simulink model "Simulink_drone_BO"  (R2025b)
settings: Solver=FixedStepAuto  StartTime=0.0  StopTime=10.0  FixedStep=dt_realtime  RelTol=1e-3
undefined symbols (not defined in the file): bool, dt_realtime, sysBO, x_init
libraries: sim3dlib x1, uavsim3dlib x1, aerolibanimutils x1
settings Model: Creator=pierr  LastModifiedBy=pierr

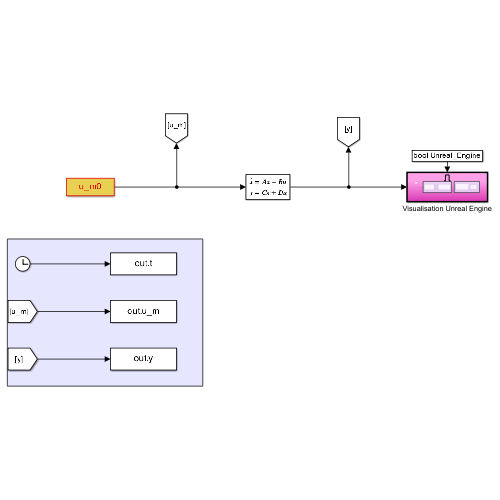
[thumbnail: Simulink's stored preview of the top-level diagram]
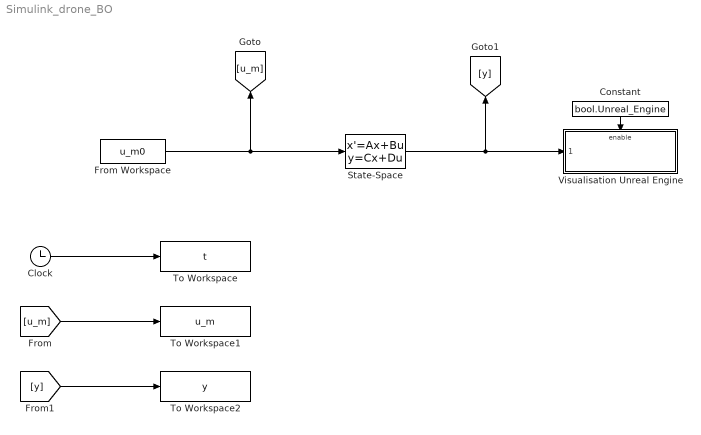
== system Simulink_drone_BO ==
  Clock : Clock
  Constant : Constant  Value=bool.Unreal_Engine
  From Workspace : FromWorkspace  VariableName=u_m0
  State-Space : StateSpace  A=sysBO.A  B=sysBO.B  C=sysBO.C  D=sysBO.D  InitialCondition=x_init
  To Workspace : ToWorkspace  VariableName=t  SaveFormat=Timeseries  SampleTime=-1
  To Workspace1 : ToWorkspace  VariableName=u_m  SaveFormat=Timeseries  SampleTime=-1
  To Workspace2 : ToWorkspace  VariableName=y  SaveFormat=Timeseries  SampleTime=-1
  Visualisation Unreal Engine : Subsystem
  wires:
  From Workspace/1 -> [u_m], State-Space/1
  Clock/1 -> To Workspace/1
  [u_m] -> To Workspace1/1
  State-Space/1 -> Visualisation Unreal Engine/1(" "), [y]
  Constant/1 -> Visualisation Unreal Engine/Enable
  [y] -> To Workspace2/1

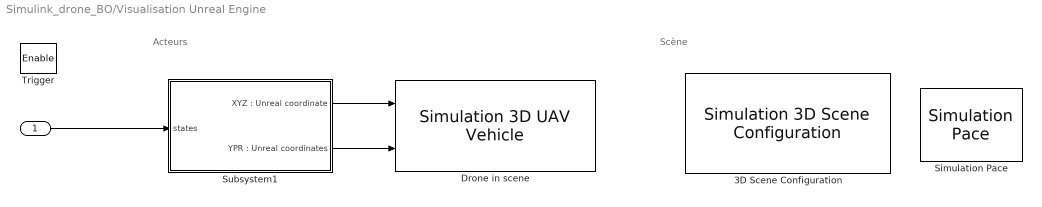
== system Simulink_drone_BO/Visualisation Unreal Engine ==
  note: Acteurs
  note: Scène
  " " : Inport
  Trigger : EnablePort
  3D Scene Configuration : sim3dlib/Simulation 3D Scene Configuration  Priority=0  ProjectFormat=Default Scenes  SceneDesc=US city block  ProjectName=C:\Program Files\MATLAB\R2025b\toolbox\shared\sim3d_projects\automotive_project_windows\UE\WindowsNoEditor\VehicleSimulation.exe  ScenePath=/Game/Maps/USCityBlock  EnableOpenDRIVE=off  vehTagList={'Custom';'Scene Origin';'donnez_moi_un_nom'}  vehTag=donnez_moi_un_nom  AttachedCameraRelativeTranslation=[0 0 0]  FreeCameraDefaultInitialTranslation=[-6, 0, 2]  AttachedCameraRelativeRotation=[0 0 0]  FreeCameraDefaultInitialRotation=[0, -15, 0]  ViewpointName=Custom  FreeCameraInitialTranslation=[0 0 0]  ViewpointTranslation=[0 0 0]  FreeCameraInitialRotation=[0 0 0]  ViewpointRotation=[0 0 0]  OpVisEn=off  Ts=dt_realtime  EnableWindow=on  EnableRemoteAccess=off  EnableWeather=off  SunAzimuth=90  SunAltitude=40.0  EnableGeospatialSun=off  Latitude=0  Longitude=0  Date=2023-01-01  Time=10:30:00  GeoTimeZone=-5.0  SunDaylightSaving=off  wind=1  clouds=10  EnableVolumetricClouds=off  CloudCoverage=0  CloudAltitude=6  fog=0  rain=0  RaindropsEffect=off  SnowDensity=0  EnableGeospatial=off  TilesetSource=Earth terrain  UseTrueOrigin=off  OriginHeight=200  OriginLatitude=40.744652  OriginLongitude=-73.988864  MapStyle=Aerial  AdditionalAssetIDs=[]  UseAdvancedSunSky=off  SolarTime=11  TimeZone=-5  Day=21  Month=9  Year=2022  UseDaylightSavingTime=on  DSTStartDay=10  DSTStartMonth=3  DSTEndDay=3  DSTEndMonth=11  DSTSwitchHour=2  sensorTag=MainCamera1  sensorId=1  sensorName=MainCamera1  mountLoc=Origin  offsetFlag=off  tmountOffset=[0, 0, 0]  rmountOffset=[0, 0, 0]  HorizontalResolution=1280  VerticalResolution=720  HorizontalFOV=60  mountPoint=[0 0 0]  mountOrientation=[0 0 0]  aMode=4  ID=1  GeoTrigger=Inactive  ViewNameList={'Custom'}  ViewTranslationList={'[0 0 0]'}  ViewRotationList={'[0 0 0]'}
      settings: LibrarySourceBlock=uavsim3dlib/Simulation 3D Scene Configuration
  Drone in scene : uavsim3dlib/Simulation 3D UAV Vehicle  Priority=-1  Mesh=Quadrotor  MeshPath=/MathWorksUAVContent/UAVs/HexaRotorUAV/HexaRotor.HexaRotor  Color=Black  ActorName=donnez_moi_un_nom  UseGlobalFrame=off  InitialTranslation=[0 0 0]  InitialRotation=[0 0 0]  InitialTranslationGlobal=[0 0 0]  InitialGeoOrigin=[0 0 0]  InitialRotationGlobal=[0 0 0]  SampleTime=-1  ActorType=SimulinkVehicle  ID=C  aMode=4  ActorTag=donnez_moi_un_nom
  Simulation Pace : aerolibanimutils/Simulation Pace  SimulationPace=1  SleepMode=Auto  OutputPaceError=off  SampleTime=dt_realtime
  Subsystem1 : Subsystem
  wires:
  " "/1 -> Subsystem1/1(states)
  Subsystem1/1("XYZ : Unreal coordinate") -> Drone in scene/1
  Subsystem1/2("YPR : Unreal coordinates") -> Drone in scene/2

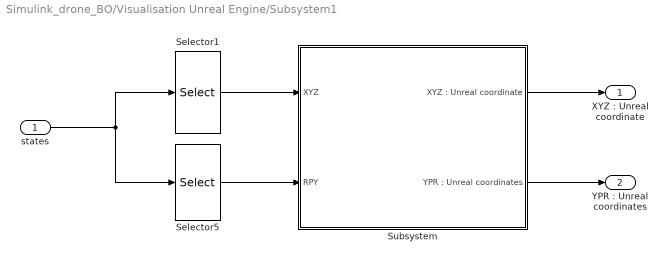
== system Simulink_drone_BO/Visualisation Unreal Engine/Subsystem1 ==
  states : Inport
  Selector1 : Selector  InputPortWidth=12  IndexOptions=Index vector (dialog)  Indices=[1 3 5]  OutputSizes=1
  Selector5 : Selector  InputPortWidth=12  IndexOptions=Index vector (dialog)  Indices=[7 9 11]  OutputSizes=1
  Subsystem : Subsystem
  "XYZ : Unreal coordinate" : Outport
  "YPR : Unreal coordinates" : Outport  Port=2
  wires:
  states/1 -> Selector1/1, Selector5/1
  Subsystem/1("XYZ : Unreal coordinate") -> "XYZ : Unreal coordinate"/1
  Selector5/1 -> Subsystem/2(RPY)
  Subsystem/2("YPR : Unreal coordinates") -> "YPR : Unreal coordinates"/1
  Selector1/1 -> Subsystem/1(XYZ)

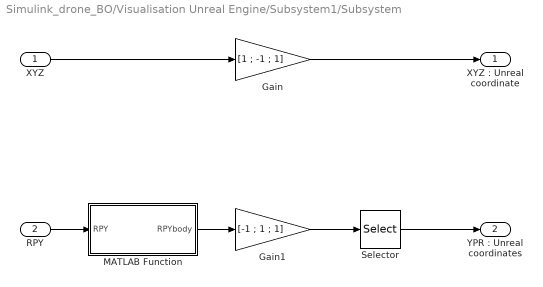
== system Simulink_drone_BO/Visualisation Unreal Engine/Subsystem1/Subsystem ==
  XYZ : Inport
  RPY : Inport  Port=2
  Gain : Gain  Gain=[1 ; -1 ; 1]
  Gain1 : Gain  Gain=[-1 ; 1 ; 1]
  MATLAB Function : MATLAB Function  TreatAsAtomicUnit=on
  Selector : Selector  InputPortWidth=3  IndexOptions=Index vector (dialog)  Indices=[3 2 1]  OutputSizes=1
  "XYZ : Unreal coordinate" : Outport
  "YPR : Unreal coordinates" : Outport  Port=2
  wires:
  Gain1/1 -> Selector/1
  RPY/1 -> MATLAB Function/1(RPY)
  MATLAB Function/1(RPYbody) -> Gain1/1
  Selector/1 -> "YPR : Unreal coordinates"/1
  XYZ/1 -> Gain/1
  Gain/1 -> "XYZ : Unreal coordinate"/1

== matlab function Simulink_drone_BO/Visualisation Unreal Engine/Subsystem1/Subsystem/MATLAB Function ==
  data: RPY input; RPYbody output
function RPYbody = fcn(RPY)


RX = [[1 0 0];...
       [0 cos(RPY(1)) -sin(RPY(1))];...
       [0 sin(RPY(1)) cos(RPY(1))]];

RY = [[cos(RPY(2)) 0 sin(RPY(2))];...
       [0 1 0];...
       [-sin(RPY(2)) 0 cos(RPY(2))]];

RZ = [[cos(RPY(3)) -sin(RPY(3)) 0];...
       [sin(RPY(3)) cos(RPY(3)) 0];...
       [0 0 1]];

RPYbody = inv(RZ*RY*RX)*RPY;
